simulink model "relay_w_positive_feedback"  (R2015a)
settings: Solver=ode45  StartTime=0.0  StopTime=200  RelTol=1e-3
values from neighbouring files (symbols this model uses):
  b = 1    [testing_relay_plant_positive_feedback.m]
  d = 1    [testing_relay_plant_positive_feedback.m]
settings Model: Creator=ra428  LastModifiedBy=ra428

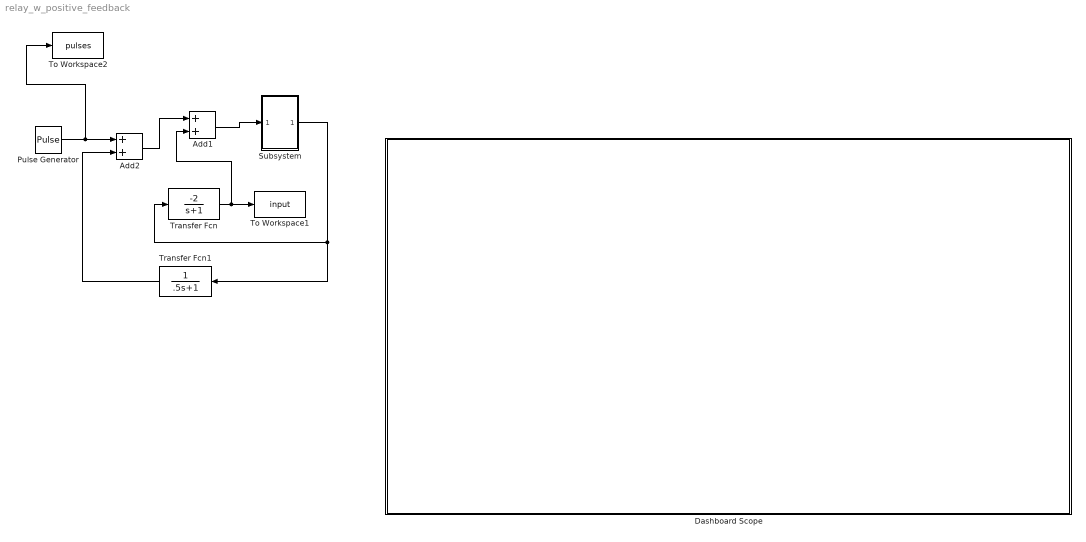
== system relay_w_positive_feedback ==
  Add1 : Sum
  Add2 : Sum
  Dashboard Scope : Subsystem  DialogController=hmiCreateDDGDialog  IsWebBlock=on  mask(MathWorksWebBlock){webBlockId=4b2ea97f-dbcc-4152-9b11-5e345150a749, webBlockType=sdiscope, ShowInitialText=on, HMISrcModelName=relay_w_positive_feedback}
      mask prompts: webBlockId "WebBlock Id"; webBlockType "WebBlock Type"; HMISrcModelName "Source Model"
      mask Help: helpview([docroot '/mapfiles/simulink.map'], 'hmi_scope')
      mask Display:
      | if strcmp(get_param(bdroot(gcb),'BlockDiagramType'), 'library')
      |     image([(matlabroot) '/toolbox/simulink/hmi/icons/DashboardScope.png']);
      | end
  Pulse Generator : DiscretePulseGenerator  PulseType=Time based  Period=200  PulseWidth=50  PhaseDelay=100
  Subsystem : Subsystem
  To Workspace1 : ToWorkspace  VariableName=input  SaveFormat=Timeseries  SampleTime=-1
  To Workspace2 : ToWorkspace  VariableName=pulses  SaveFormat=Timeseries  SampleTime=-1
  Transfer Fcn : TransferFcn  Numerator=[-2]  Denominator=[1 1]
  Transfer Fcn1 : TransferFcn  Denominator=[.5 1]
  wires:
  Transfer Fcn/1 -> Add1/2, To Workspace1/1
  Pulse Generator/1 -> Add2/1, To Workspace2/1
  Transfer Fcn1/1 -> Add2/2
  Add2/1 -> Add1/1
  Subsystem/1(Out1) -> Transfer Fcn1/1, Transfer Fcn/1
  Add1/1 -> Subsystem/1(In2)

== system relay_w_positive_feedback/Dashboard Scope ==

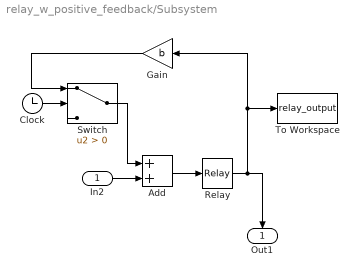
== system relay_w_positive_feedback/Subsystem ==
  In2 : Inport
  Add : Sum
  Clock : Clock
  Gain : Gain  Gain=b
  Relay : Relay  OnSwitchValue=0  OffSwitchValue=0  OnOutputValue=d  OffOutputValue=-d
  Switch : Switch  Criteria=u2 > Threshold
  To Workspace : ToWorkspace  VariableName=relay_output  SaveFormat=Timeseries  SampleTime=-1
  Out1 : Outport
  wires:
  Clock/1 -> Switch/2
  ? -> Switch/3
  Gain/1 -> Switch/1
  In2/1 -> Add/2
  Relay/1 -> Out1/1, To Workspace/1, Gain/1
  Switch/1 -> Add/1
  Add/1 -> Relay/1
